simulink model "mutia"  (R2017a)
settings: Solver=VariableStepAuto  StartTime=0.0  StopTime=10.0  RelTol=1e-3
undefined symbols (not defined in the file): mutia
libraries: fuzblock x1
settings Model: Creator=xp  LastModifiedBy=xp

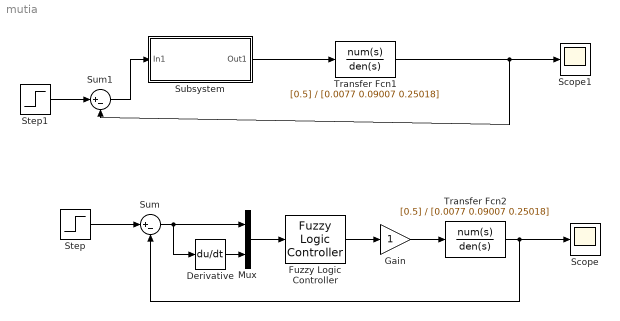
== system mutia ==
  Derivative : Derivative
  Fuzzy Logic Controller : fuzblock/Fuzzy Logic  Controller  fis=[mutia]
  Gain : Gain
  Mux : Mux  Inputs=2
  Scope : Scope
  Scope1 : Scope
  Step : Step  SampleTime=0
  Step1 : Step  SampleTime=0
  Subsystem : Subsystem
  Sum : Sum  Inputs=|+-
  Sum1 : Sum  Inputs=|+-
  Transfer Fcn1 : TransferFcn  Numerator=[0.5]  Denominator=[0.0077 0.09007 0.25018]
  Transfer Fcn2 : TransferFcn  Numerator=[0.5]  Denominator=[0.0077 0.09007 0.25018]
  wires:
  Step/1 -> Sum/1
  Sum/1 -> Derivative/1, Mux/1
  Derivative/1 -> Mux/2
  Mux/1 -> Fuzzy Logic Controller/1
  Fuzzy Logic Controller/1 -> Gain/1
  Gain/1 -> Transfer Fcn2/1
  Transfer Fcn2/1 -> Scope/1, Sum/2
  Step1/1 -> Sum1/1
  Sum1/1 -> Subsystem/1(In1)
  Subsystem/1(Out1) -> Transfer Fcn1/1
  Transfer Fcn1/1 -> Sum1/2, Scope1/1

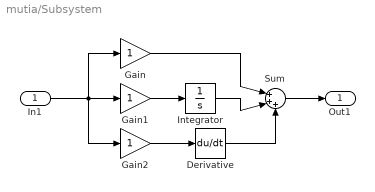
== system mutia/Subsystem ==
  In1 : Inport
  Derivative : Derivative
  Gain : Gain
  Gain1 : Gain
  Gain2 : Gain
  Integrator : Integrator
  Sum : Sum  Inputs=|+++
  Out1 : Outport
  wires:
  In1/1 -> Gain2/1, Gain/1, Gain1/1
  Gain1/1 -> Integrator/1
  Integrator/1 -> Sum/2
  Gain/1 -> Sum/1
  Gain2/1 -> Derivative/1
  Derivative/1 -> Sum/3
  Sum/1 -> Out1/1
